simulink model "Measure_BH_curve3"  (R2016a)
settings: Solver=ode23tb  StartTime=0.0  StopTime=0.1  RelTol=1e-3
undefined symbols (not defined in the file or in its folder): i
libraries: powerlib x7
settings Model: Creator=Administrator  LastModifiedBy=Administrator
settings DataIOCC: LimitDataPoints=on  SaveFormat=Array
settings DebuggingCC: SolverPrmCheckMsg=warning
settings HardwareCC: ProdBitPerPointer=32  ProdLargestAtomicFloat=None  ProdIntDivRoundTo=Undefined  ProdEndianess=Unspecified  ProdWordSize=32  ProdHWDeviceType=32-bit Generic
settings ModelReferenceCC: PropagateSignalLabelsOutOfModel=off
settings ConfigComp: CovModelRefEnable=Off  CovSFcnEnable=off

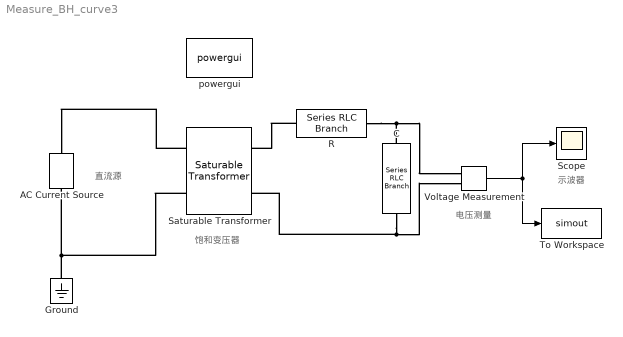
== system Measure_BH_curve3 ==
  note: 示波器
  note: 电压测量
  note: 饱和变压器
  note: 直流源
  AC Current Source : powerlib/Electrical Sources/AC Current Source  Amplitude=i  Phase=90  Frequency=0  SampleTime=0  Measurements=None
  C : powerlib/Elements/Series RLC Branch  LConnTagsString=__new0  RConnTagsString=__new0  BranchType=C  Resistance=1  Inductance=1e-3  SetiL0=off  InitialCurrent=0  Capacitance=10e-6  Setx0=off  InitialVoltage=0  Measurements=None
  Ground : powerlib/Elements/Ground  LConnTagsString=a
  R : powerlib/Elements/Series RLC Branch  LConnTagsString=__new0  RConnTagsString=__new0  BranchType=R  Resistance=470e3  Inductance=1e-3  SetiL0=off  InitialCurrent=0  Capacitance=1e-6  Setx0=off  InitialVoltage=0  Measurements=None
  Saturable Transformer : powerlib/Elements/Saturable Transformer  ThreeWindings=off  Hysteresis=off  DataFile='my_hysteresis.mat'  Measurements=None  UNITS=pu  NominalPower=[250e6 60]  Winding1=[7.35e+05 0.002 0]  Winding2=[3.15e+05 0.002 0.08]  Winding3=[3.15e+05 0.002 0.08]  Saturation=[0 0;0.0024001 1.2;1 1.5201]  CoreLoss=500.02  MoreParameters=off  BreakLoop=off  DataType=off  InitialFlux=0  TransfoNumber=1
  Scope : Scope
  To Workspace : ToWorkspace  VariableName=simout  SaveFormat=Timeseries  SampleTime=-1
  Voltage Measurement : powerlib/Measurements/Voltage Measurement  PhasorSimulation=off  OutputType=Complex  PSBequivalent=0
  powergui : powerlib/powergui  Priority=1  SimulationMode=Discrete  SolverType=Tustin/Backward Euler (TBE)  SampleTime=50e-6  frequency=60  SPID=off  DisableSnubberDevices=off  DisableRonSwitches=off  DisableVfSwitches=off  SwTol=0  DisplayEquations=off  Interpol=off  ExternalGateDelay=off  methode=off  Ts=10  FunctionMessages=off  echomessages=off  HookPort=off  EnableUseOfTLC=off  x0status=blocks  frequencyindice=0  Pbase=100e6  ErrMax=1e-4  Iterations=50  UnitsV=kV  UnitsW=MW  buscounter=0  RestoreLinks=warning  ResistiveCurrentMeasurement=off  Frange=[0:2:500]  Ylog=off  Xlog=on  ShowGrid=off  save=off  variable=ZData  structure=0  ZoomFFT=off  StartTime=0.0  cycles=1  DisplayStyle=1  fundamental=60  FreqAxis=off  MaxFrequency=1000  frequencyindicesteady=1  RmsSteady=1  display=off
  wires:
  Voltage Measurement/1 -> To Workspace/1, Scope/1
  connections:
  C/RConn1 -- Saturable Transformer/RConn2 -- Voltage Measurement/LConn2
  Saturable Transformer/LConn2 -- AC Current Source/LConn1 -- Ground/LConn1
  R/RConn1 -- Voltage Measurement/LConn1 -- C/LConn1
  Saturable Transformer/LConn1 -- AC Current Source/RConn1
  R/LConn1 -- Saturable Transformer/RConn1
